simulink model "vymennik5cviko"  (R2019b)
settings: Solver=VariableStepAuto  StartTime=0.0  StopTime=1  RelTol=1e-3
values from neighbouring files (symbols this model uses):
  cpr = 4186    [cv5par.m]
  l12r = 1.02e6    (= 1020000)    [cv5par.m]
  M1r = 500    [cv5par.m]
  M2r = 500    [cv5par.m]
  ror = 1000    [cv5par.m]
  S1r = 1.885    [cv5par.m]
  Ti1r = 90    [cv5par.m]
  Ti2r = 20    [cv5par.m]
  V1r = 0.05    [cv5par.m]
  V2r = 0.0283    [cv5par.m]
settings Model: Creator=student  LastModifiedBy=student

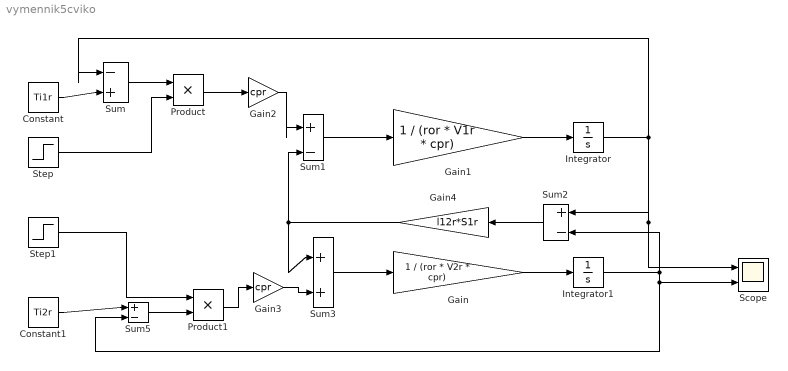
== system vymennik5cviko ==
  Constant : Constant  Value=Ti1r
  Constant1 : Constant  Value=Ti2r
  Gain : Gain  Gain=1 / (ror * V2r * cpr)
  Gain1 : Gain  Gain=1 / (ror * V1r * cpr)
  Gain2 : Gain  Gain=cpr
  Gain3 : Gain  Gain=cpr
  Gain4 : Gain  Gain=l12r*S1r
  Integrator : Integrator  InitialCondition=20
  Integrator1 : Integrator  InitialCondition=20
  Product : Product
  Product1 : Product
  Scope : Scope  NumInputPorts=2
  Step : Step  Time=3  Before=M1r  After=M1r/2  SampleTime=0
  Step1 : Step  Time=0.5  Before=M2r  After=M2r/2  SampleTime=0
  Sum : Sum  Inputs=|-+
  Sum1 : Sum  Inputs=|+-
  Sum2 : Sum  Inputs=|+-
  Sum3 : Sum  Inputs=|++
  Sum5 : Sum  Inputs=|+-
  wires:
  Constant/1 -> Sum/2
  Sum/1 -> Product/1
  Product/1 -> Gain2/1
  Gain2/1 -> Sum1/1
  Sum1/1 -> Gain1/1
  Gain1/1 -> Integrator/1
  Integrator/1 -> Scope/1, Sum2/1, Sum/1
  Step/1 -> Product/2
  Sum2/1 -> Gain4/1
  Gain4/1 -> Sum3/1, Sum1/2
  Sum3/1 -> Gain/1
  Gain/1 -> Integrator1/1
  Integrator1/1 -> Sum5/2, Scope/2, Sum2/2
  Constant1/1 -> Sum5/1
  Sum5/1 -> Product1/2
  Step1/1 -> Product1/1
  Product1/1 -> Gain3/1
  Gain3/1 -> Sum3/2
